simulink model "PeakDetect_500"  (R2018b)
settings: Solver=FixedStepAuto  StartTime=0  StopTime=500*(15e-9)  FixedStep=15e-9  RelTol=1e-3
libraries: simulink x35, hdlsllib x34
(part 2 of 3)

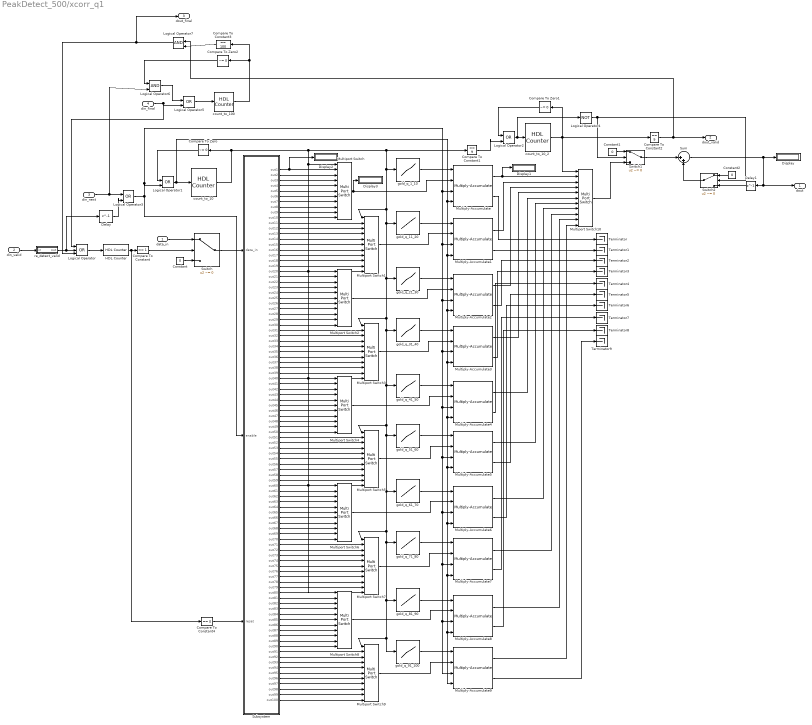
== system PeakDetect_500/xcorr_q1 ==
  data_in : Inport  OutDataTypeStr=fixdt(1,16,15)
  din_valid : Inport  Port=2
  din_next : Inport  Port=3
  din_final : Inport  Port=4
  Compare To Constant : simulink/Logic and Bit Operations/Compare To Constant  relop===  const=1  OutDataTypeStr=boolean
  Compare To Constant1 : simulink/Logic and Bit Operations/Compare To Constant  relop===  const=9  OutDataTypeStr=boolean
  Compare To Constant2 : simulink/Logic and Bit Operations/Compare To Constant  relop===  const=9  OutDataTypeStr=boolean
  Compare To Constant3 : simulink/Logic and Bit Operations/Compare To Constant  relop===  const=100  OutDataTypeStr=boolean
  Compare To Constant4 : simulink/Logic and Bit Operations/Compare To Constant  relop===  const=0  OutDataTypeStr=boolean
  Compare To Zero : simulink/Logic and Bit Operations/Compare To Zero  relop=~=  OutDataTypeStr=boolean
  Compare To Zero1 : simulink/Logic and Bit Operations/Compare To Zero  relop=~=  OutDataTypeStr=boolean
  Compare To Zero2 : simulink/Logic and Bit Operations/Compare To Zero  relop=~=  OutDataTypeStr=boolean
  Constant : Constant  Value=0  OutDataTypeStr=fixdt(1,16,15)  SampleTime=-1
  Constant1 : Constant  Value=0  OutDataTypeStr=Inherit: Inherit via back propagation  SampleTime=-1
  Constant2 : Constant  Value=0  OutDataTypeStr=Inherit: Inherit via back propagation  SampleTime=-1
  Delay : Delay  DelayLength=1
  Delay1 : Delay  DelayLength=1
  Display{,1..3} (4 alike) : Display
  HDL Counter : hdlsllib/Sources/HDL Counter  CountType=Count limited  CountInit=0  CountStep=1  CountMax=2  CountFromType=Initial value  CountFrom=0  CountResetPort=off  CountLoadPort=off  CountEnbPort=on  CountDirPort=off  CountDataType=Unsigned  CountWordLen=8  CountFracLen=0  CountSampTime=1
      settings: SourceProductBaseCode=HD
  Logical Operator : Logic  Operator=OR  Inputs=3  IconShape=distinctive  AllPortsSameDT=off  OutDataTypeStr=boolean
  Logical Operator{1..3,5} (4 alike) : Logic  Operator=OR  IconShape=distinctive  AllPortsSameDT=off  OutDataTypeStr=boolean
  Logical Operator4 : Logic  Operator=NOT  IconShape=distinctive  AllPortsSameDT=off  OutDataTypeStr=boolean
  Logical Operator6 : Logic  IconShape=distinctive  AllPortsSameDT=off  OutDataTypeStr=boolean
  Logical Operator7 : Logic  IconShape=distinctive  AllPortsSameDT=off  OutDataTypeStr=boolean
  Multiply-Accumulate{,1..9} (10 alike) : hdlsllib/HDL Operations/Multiply-Accumulate  opMode=Streaming - using Start and End ports  initValueSetting=Dialog  initValue=0  initValueSetting2=Dialog  initValue2=0  initValueSetting3=Dialog  initValue3=0  num_samples=2  RndMeth2=Floor  RndMeth3=Floor  datatype2=fixdt(1,32,16)  datatype3=Inherit: Inherit via back propagation  validOut=on  endInandOut=off  startOut=off  countOut=on  dim=-1  DoSatur=off  parallel=off
      settings: SourceProductName=HDL Coder  SourceProductBaseCode=HD
  Multiport Switch{,1..9} (10 alike) : MultiPortSwitch  DataPortOrder=Zero-based contiguous  Inputs=10  zeroidx=on  OutDataTypeStr=fixdt(1,16,15)
  Multiport Switch10 : MultiPortSwitch  DataPortOrder=Zero-based contiguous  Inputs=10  zeroidx=on  OutDataTypeStr=fixdt(1,32,16)
  Subsystem : Subsystem
  Sum : Sum  Inputs=|++  OutDataTypeStr=Inherit: Inherit via back propagation
  Switch : Switch  Criteria=u2 ~= 0  OutDataTypeStr=Inherit: Inherit via back propagation
  Switch1 : Switch  Criteria=u2 ~= 0  OutDataTypeStr=Inherit: Inherit via back propagation
  Switch2 : Switch  Criteria=u2 ~= 0  OutDataTypeStr=Inherit: Inherit via back propagation
  Terminator{,1..9} (10 alike) : Terminator
  count_to_10 : hdlsllib/Sources/HDL Counter  CountType=Count limited  CountInit=0  CountStep=1  CountMax=9  CountFromType=Initial value  CountFrom=0  CountResetPort=off  CountLoadPort=off  CountEnbPort=on  CountDirPort=off  CountDataType=Unsigned  CountWordLen=4  CountFracLen=0  CountSampTime=1
      settings: SourceProductBaseCode=HD
  count_to_100 : hdlsllib/Sources/HDL Counter  CountType=Count limited  CountInit=0  CountStep=1  CountMax=100  CountFromType=Initial value  CountFrom=0  CountResetPort=off  CountLoadPort=off  CountEnbPort=on  CountDirPort=off  CountDataType=Unsigned  CountWordLen=8  CountFracLen=0  CountSampTime=1
      settings: SourceProductBaseCode=HD
  count_to_10_2 : hdlsllib/Sources/HDL Counter  CountType=Count limited  CountInit=0  CountStep=1  CountMax=9  CountFromType=Initial value  CountFrom=0  CountResetPort=off  CountLoadPort=off  CountEnbPort=on  CountDirPort=off  CountDataType=Unsigned  CountWordLen=4  CountFracLen=0  CountSampTime=1
      settings: SourceProductBaseCode=HD
  gold_q_11_20 : Lookup_n-D  NumberOfTableDimensions=1  LookupTableObject=''  BreakpointsForDimension1=uint8([0,1,2,3,4,5,6,7,8,9])  BreakpointsForDimension1FirstPoint=10  BreakpointsForDimension2FirstPoint=10  BreakpointsForDimension1Spacing=12  BreakpointsForDimension2Spacing=12  IndexSearchMethod=Evenly spaced points  Table=|  TableDataTypeStr=fixdt(1,16,15)  InterpMethod=Flat  DiagnosticForOutOfRangeInput=Error  InternalRulePriority=Speed  OutDataTypeStr=fixdt(1,16,15)  RndMeth=Simplest  InputSameDT=on
      | -1*[0.236906374990369
      | 0.265062589296935
      | 0.290853922757751
      | 0.306866645010829
      | 0.306877356493505
      | 0.282583044796408
      | 0.237895318583737
      | 0.179451570247324
      | 0.106711739895776
      | 0.0250742736874029]
  gold_q_1_10 : Lookup_n-D  NumberOfTableDimensions=1  LookupTableObject=''  BreakpointsForDimension1=uint8([0,1,2,3,4,5,6,7,8,9])  BreakpointsForDimension1FirstPoint=10  BreakpointsForDimension2FirstPoint=10  BreakpointsForDimension1Spacing=12  BreakpointsForDimension2Spacing=12  IndexSearchMethod=Evenly spaced points  Table=|  TableDataTypeStr=fixdt(1,16,15)  InterpMethod=Flat  DiagnosticForOutOfRangeInput=Error  InternalRulePriority=Speed  OutDataTypeStr=fixdt(1,16,15)  RndMeth=Simplest  InputSameDT=on
      | -1*[0.357169275362262
      | 0.373691122276015
      | 0.363136475782144
      | 0.332586509539436
      | 0.291374087870011
      | 0.249422279627694
      | 0.215579045674242
      | 0.200455944131647
      | 0.201796906991478
      | 0.213779029408702]
  gold_q_21_30 : Lookup_n-D  NumberOfTableDimensions=1  LookupTableObject=''  BreakpointsForDimension1=uint8([0,1,2,3,4,5,6,7,8,9])  BreakpointsForDimension1FirstPoint=10  BreakpointsForDimension2FirstPoint=10  BreakpointsForDimension1Spacing=12  BreakpointsForDimension2Spacing=12  IndexSearchMethod=Evenly spaced points  Table=|  TableDataTypeStr=fixdt(1,16,15)  InterpMethod=Flat  DiagnosticForOutOfRangeInput=Error  InternalRulePriority=Speed  OutDataTypeStr=fixdt(1,16,15)  RndMeth=Simplest  InputSameDT=on
      | -1*[-0.0591515848508664
      | -0.139598314313151
      | -0.210629837752387
      | -0.263713716480122
      | -0.301489962058033
      | -0.328238114626508
      | -0.340130412877520
      | -0.338689881672749
      | -0.326243180584237
      | -0.305614110780615]
  gold_q_31_40 : Lookup_n-D  NumberOfTableDimensions=1  LookupTableObject=''  BreakpointsForDimension1=uint8([0,1,2,3,4,5,6,7,8,9])  BreakpointsForDimension1FirstPoint=10  BreakpointsForDimension2FirstPoint=10  BreakpointsForDimension1Spacing=12  BreakpointsForDimension2Spacing=12  IndexSearchMethod=Evenly spaced points  Table=|  TableDataTypeStr=fixdt(1,16,15)  InterpMethod=Flat  DiagnosticForOutOfRangeInput=Error  InternalRulePriority=Speed  OutDataTypeStr=fixdt(1,16,15)  RndMeth=Simplest  InputSameDT=on
      | -1*[-0.279858098355888
      | -0.247814863771713
      | -0.225446174923891
      | -0.202743193363060
      | -0.186527042991191
      | -0.178781266249413
      | -0.180711431323688
      | -0.192575241083779
      | -0.213551675353351
      | -0.245925394077466]
  gold_q_41_50 : Lookup_n-D  NumberOfTableDimensions=1  LookupTableObject=''  BreakpointsForDimension1=uint8([0,1,2,3,4,5,6,7,8,9])  BreakpointsForDimension1FirstPoint=10  BreakpointsForDimension2FirstPoint=10  BreakpointsForDimension1Spacing=12  BreakpointsForDimension2Spacing=12  IndexSearchMethod=Evenly spaced points  Table=|  TableDataTypeStr=fixdt(1,16,15)  InterpMethod=Flat  DiagnosticForOutOfRangeInput=Error  InternalRulePriority=Speed  OutDataTypeStr=fixdt(1,16,15)  RndMeth=Simplest  InputSameDT=on
      | -1*[-0.273649789754997
      | -0.305507933389466
      | -0.332526349511340
      | -0.349961882407133
      | -0.353614169955030
      | -0.340366684130075
      | -0.308641627170326
      | -0.254460428744123
      | -0.185247665828561
      | -0.110080691949015]
  gold_q_51_60 : Lookup_n-D  NumberOfTableDimensions=1  LookupTableObject=''  BreakpointsForDimension1=uint8([0,1,2,3,4,5,6,7,8,9])  BreakpointsForDimension1FirstPoint=10  BreakpointsForDimension2FirstPoint=10  BreakpointsForDimension1Spacing=12  BreakpointsForDimension2Spacing=12  IndexSearchMethod=Evenly spaced points  Table=|  TableDataTypeStr=fixdt(1,16,15)  InterpMethod=Flat  DiagnosticForOutOfRangeInput=Error  InternalRulePriority=Speed  OutDataTypeStr=fixdt(1,16,15)  RndMeth=Simplest  InputSameDT=on
      | -1*[-0.0297558495000079
      | 0.0499350486257353
      | 0.122950591883728
      | 0.183532283875116
      | 0.226715241693549
      | 0.244522518247979
      | 0.247772413924009
      | 0.223279362418140
      | 0.176793915855740
      | 0.111355596734925]
  gold_q_61_70 : Lookup_n-D  NumberOfTableDimensions=1  LookupTableObject=''  BreakpointsForDimension1=uint8([0,1,2,3,4,5,6,7,8,9])  BreakpointsForDimension1FirstPoint=10  BreakpointsForDimension2FirstPoint=10  BreakpointsForDimension1Spacing=12  BreakpointsForDimension2Spacing=12  IndexSearchMethod=Evenly spaced points  Table=|  TableDataTypeStr=fixdt(1,16,15)  InterpMethod=Flat  DiagnosticForOutOfRangeInput=Error  InternalRulePriority=Speed  OutDataTypeStr=fixdt(1,16,15)  RndMeth=Simplest  InputSameDT=on
      | -1*[0.0312880626224120
      | -0.0580988665112754
      | -0.150830519884918
      | -0.236354458852815
      | -0.321361371110983
      | -0.387151947785857
      | -0.432910784333285
      | -0.454553321854592
      | -0.449340647995131
      | -0.416266380216616]
  gold_q_71_80 : Lookup_n-D  NumberOfTableDimensions=1  LookupTableObject=''  BreakpointsForDimension1=uint8([0,1,2,3,4,5,6,7,8,9])  BreakpointsForDimension1FirstPoint=10  BreakpointsForDimension2FirstPoint=10  BreakpointsForDimension1Spacing=12  BreakpointsForDimension2Spacing=12  IndexSearchMethod=Evenly spaced points  Table=|  TableDataTypeStr=fixdt(1,16,15)  InterpMethod=Flat  DiagnosticForOutOfRangeInput=Error  InternalRulePriority=Speed  OutDataTypeStr=fixdt(1,16,15)  RndMeth=Simplest  InputSameDT=on
      | -1*[-0.356405677154333
      | -0.268905527196357
      | -0.172503144328213
      | -0.0623088722264564
      | 0.0478292512438748
      | 0.147701871156711
      | 0.227579808283800
      | 0.279365016179912
      | 0.297653875710056
      | 0.276310228166542]
  gold_q_81_90 : Lookup_n-D  NumberOfTableDimensions=1  LookupTableObject=''  BreakpointsForDimension1=uint8([0,1,2,3,4,5,6,7,8,9])  BreakpointsForDimension1FirstPoint=10  BreakpointsForDimension2FirstPoint=10  BreakpointsForDimension1Spacing=12  BreakpointsForDimension2Spacing=12  IndexSearchMethod=Evenly spaced points  Table=|  TableDataTypeStr=fixdt(1,16,15)  InterpMethod=Flat  DiagnosticForOutOfRangeInput=Error  InternalRulePriority=Speed  OutDataTypeStr=fixdt(1,16,15)  RndMeth=Simplest  InputSameDT=on
      | -1*[0.222595237130309
      | 0.147485843722747
      | 0.0555170073150737
      | -0.0424496465550990
      | -0.134707118174198
      | -0.210100315272752
      | -0.259403813850479
      | -0.272248751146779
      | -0.259403813850479
      | -0.210100315272752]
  gold_q_91_100 : Lookup_n-D  NumberOfTableDimensions=1  LookupTableObject=''  BreakpointsForDimension1=uint8([0,1,2,3,4,5,6,7,8,9])  BreakpointsForDimension1FirstPoint=10  BreakpointsForDimension2FirstPoint=10  BreakpointsForDimension1Spacing=12  BreakpointsForDimension2Spacing=12  IndexSearchMethod=Evenly spaced points  Table=|  TableDataTypeStr=fixdt(1,16,15)  InterpMethod=Flat  DiagnosticForOutOfRangeInput=Error  InternalRulePriority=Speed  OutDataTypeStr=fixdt(1,16,15)  RndMeth=Simplest  InputSameDT=on
      | -1*[-0.134707118174198
      | -0.0424496465550989
      | 0.0555170073150737
      | 0.147485843722747
      | 0.222595237130309
      | 0.267820298855522
      | 0.290378842162360
      | 0.275261187855880
      | 0.228204197191429
      | 0.153805243290024]
  re_detect_valid : Subsystem
  dout : Outport  OutDataTypeStr=fixdt(1,32,16)
  dout_valid : Outport  Port=2
  dout_final : Outport  Port=3
  wires:
  Subsystem/63(out63) -> Multiport Switch6/4
  Subsystem/83(out83) -> Multiport Switch8/4
  Subsystem/87(out87) -> Multiport Switch8/8
  Subsystem/57(out57) -> Multiport Switch5/8
  count_to_10/1 -> Compare To Zero/1, Multiport Switch8/1, Multiport Switch6/1, Multiport Switch4/1, Multiport Switch2/1, Multiport Switch/1, gold_q_11_20/1, gold_q_21_30/1, gold_q_31_40/1, gold_q_41_50/1, gold_q_51_60/1, gold_q_61_70/1, gold_q_71_80/1, gold_q_81_90/1, gold_q_91_100/1, Multiport Switch9/1, Multiport Switch7/1, Multiport Switch5/1, Multiport Switch3/1, Multiport Switch1/1, gold_q_1_10/1, Compare To Constant1/1
  Subsystem/97(out97) -> Multiport Switch9/8
  Multiply-Accumulate4/1 -> Multiport Switch10/6
  Subsystem/65(out65) -> Multiport Switch6/6
  Subsystem/99(out99) -> Multiport Switch9/10
  Subsystem/73(out73) -> Multiport Switch7/4
  Subsystem/49(out49) -> Multiport Switch4/10
  Multiply-Accumulate/2 -> Terminator/1
  din_final/1 -> Logical Operator/1, Logical Operator5/2
  count_to_10_2/1 -> Compare To Constant2/1, Multiport Switch10/1, Compare To Zero1/1
  Multiport Switch8/1 -> Multiply-Accumulate8/2
  Compare To Constant2/1 -> dout_valid/1, Logical Operator7/1
  Subsystem/61(out61) -> Multiport Switch6/2
  Subsystem/28(out28) -> Multiport Switch2/9
  Subsystem/1(out1) -> Display2/1, Multiport Switch/2
  Multiply-Accumulate6/1 -> Multiport Switch10/8
  Subsystem/100(out100) -> Multiport Switch9/11
  Logical Operator/1 -> HDL Counter/1
  din_valid/1 -> re_detect_valid/1(in)
  Subsystem/68(out68) -> Multiport Switch6/9
  Subsystem/56(out56) -> Multiport Switch5/7
  Subsystem/13(out13) -> Multiport Switch1/4
  Subsystem/67(out67) -> Multiport Switch6/8
  Subsystem/66(out66) -> Multiport Switch6/7
  Logical Operator2/1 -> Logical Operator4/1, count_to_10_2/1
  Constant/1 -> Switch/3
  Compare To Zero/1 -> Logical Operator1/1
  Subsystem/89(out89) -> Multiport Switch8/10
  Multiport Switch5/1 -> Multiply-Accumulate5/2
  Subsystem/29(out29) -> Multiport Switch2/10
  Compare To Constant/1 -> Switch/2
  gold_q_91_100/1 -> Multiply-Accumulate9/1
  Subsystem/52(out52) -> Multiport Switch5/3
  re_detect_valid/1(out) -> Delay/1, Logical Operator/2
  Logical Operator1/1 -> count_to_10/1, Multiply-Accumulate2/4, Multiply-Accumulate9/4, Multiply-Accumulate8/4, Multiply-Accumulate7/4, Multiply-Accumulate6/4, Multiply-Accumulate5/4, Multiply-Accumulate4/4, Multiply-Accumulate3/4, Multiply-Accumulate1/4, Multiply-Accumulate/4
  Subsystem/76(out76) -> Multiport Switch7/7
  Sum/1 -> dout/1, Delay1/1, Display/1
  Logical Operator3/1 -> Subsystem/2(enable), Multiply-Accumulate9/3, Multiply-Accumulate8/3, Multiply-Accumulate7/3, Multiply-Accumulate6/3, Multiply-Accumulate5/3, Multiply-Accumulate4/3, Multiply-Accumulate3/3, Multiply-Accumulate2/3, Multiply-Accumulate1/3, Multiply-Accumulate/3, Logical Operator1/2
  Subsystem/2(out2) -> Multiport Switch/3
  Subsystem/88(out88) -> Multiport Switch8/9
  Subsystem/64(out64) -> Multiport Switch6/5
  Subsystem/41(out41) -> Multiport Switch4/2
  Multiply-Accumulate9/2 -> Terminator9/1
  din_next/1 -> Logical Operator6/2, Logical Operator3/1
  Subsystem/11(out11) -> Multiport Switch1/2
  Subsystem/96(out96) -> Multiport Switch9/7
  Switch1/1 -> Sum/1
  Subsystem/80(out80) -> Multiport Switch7/11
  Subsystem/54(out54) -> Multiport Switch5/5
  Subsystem/82(out82) -> Multiport Switch8/3
  Multiply-Accumulate4/2 -> Terminator4/1
  Subsystem/6(out6) -> Multiport Switch/7
  Subsystem/45(out45) -> Multiport Switch4/6
  Multiport Switch4/1 -> Multiply-Accumulate4/2
  Logical Operator4/1 -> Switch1/2, Switch2/2
  Subsystem/58(out58) -> Multiport Switch5/9
  Subsystem/81(out81) -> Multiport Switch8/2
  Subsystem/44(out44) -> Multiport Switch4/5
  Subsystem/86(out86) -> Multiport Switch8/7
  Subsystem/85(out85) -> Multiport Switch8/6
  Logical Operator5/1 -> count_to_100/1
  Multiport Switch/1 -> Multiply-Accumulate/2, Display3/1
  Subsystem/27(out27) -> Multiport Switch2/8
  gold_q_31_40/1 -> Multiply-Accumulate3/1
  Subsystem/93(out93) -> Multiport Switch9/4
  Compare To Zero1/1 -> Logical Operator2/1
  Subsystem/39(out39) -> Multiport Switch3/10
  Subsystem/84(out84) -> Multiport Switch8/5
  Subsystem/70(out70) -> Multiport Switch6/11
  Subsystem/77(out77) -> Multiport Switch7/8
  Subsystem/62(out62) -> Multiport Switch6/3
  Subsystem/95(out95) -> Multiport Switch9/6
  gold_q_1_10/1 -> Multiply-Accumulate/1
  Compare To Zero2/1 -> Logical Operator6/1
  Multiply-Accumulate1/1 -> Multiport Switch10/3
  Subsystem/47(out47) -> Multiport Switch4/8
  Multiply-Accumulate3/2 -> Terminator3/1
  Subsystem/22(out22) -> Multiport Switch2/3
  Subsystem/92(out92) -> Multiport Switch9/3
  count_to_100/1 -> Compare To Constant3/1, Compare To Zero2/1
  Multiport Switch3/1 -> Multiply-Accumulate3/2
  Subsystem/59(out59) -> Multiport Switch5/10
  Subsystem/9(out9) -> Multiport Switch/10
  Subsystem/5(out5) -> Multiport Switch/6
  gold_q_11_20/1 -> Multiply-Accumulate1/1
  data_in/1 -> Switch/1
  Subsystem/90(out90) -> Multiport Switch8/11
  Subsystem/10(out10) -> Multiport Switch/11
  Subsystem/75(out75) -> Multiport Switch7/6
  Subsystem/18(out18) -> Multiport Switch1/9
  Subsystem/12(out12) -> Multiport Switch1/3
  Subsystem/25(out25) -> Multiport Switch2/6
  Subsystem/43(out43) -> Multiport Switch4/4
  Subsystem/72(out72) -> Multiport Switch7/3
  Subsystem/30(out30) -> Multiport Switch2/11
  Subsystem/8(out8) -> Multiport Switch/9
  Subsystem/60(out60) -> Multiport Switch5/11
  HDL Counter/1 -> Compare To Constant4/1, Compare To Constant/1
  Multiply-Accumulate8/2 -> Terminator8/1
  Subsystem/17(out17) -> Multiport Switch1/8
  Multiply-Accumulate9/1 -> Multiport Switch10/11
  Subsystem/26(out26) -> Multiport Switch2/7
  Subsystem/35(out35) -> Multiport Switch3/6
  Subsystem/24(out24) -> Multiport Switch2/5
  Subsystem/20(out20) -> Multiport Switch1/11
  Subsystem/71(out71) -> Multiport Switch7/2
  Subsystem/78(out78) -> Multiport Switch7/9
  Multiport Switch9/1 -> Multiply-Accumulate9/2
  Subsystem/7(out7) -> Multiport Switch/8
  Subsystem/3(out3) -> Multiport Switch/4
  Subsystem/79(out79) -> Multiport Switch7/10
  Multiport Switch10/1 -> Switch1/3
  Subsystem/15(out15) -> Multiport Switch1/6
  Subsystem/14(out14) -> Multiport Switch1/5
  Multiply-Accumulate/1 -> Display1/1, Multiport Switch10/2
  Subsystem/42(out42) -> Multiport Switch4/3
  Subsystem/16(out16) -> Multiport Switch1/7
  Logical Operator6/1 -> Logical Operator5/1
  Logical Operator7/1 -> dout_final/1, Logical Operator/3
  Subsystem/53(out53) -> Multiport Switch5/4
  Subsystem/37(out37) -> Multiport Switch3/8
  Subsystem/55(out55) -> Multiport Switch5/6
  Subsystem/48(out48) -> Multiport Switch4/9
  Subsystem/4(out4) -> Multiport Switch/5
  Subsystem/50(out50) -> Multiport Switch4/11
  Subsystem/40(out40) -> Multiport Switch3/11
  Switch/1 -> Subsystem/1(data_in)
  Subsystem/19(out19) -> Multiport Switch1/10
  Subsystem/38(out38) -> Multiport Switch3/9
  Subsystem/33(out33) -> Multiport Switch3/4
  Subsystem/46(out46) -> Multiport Switch4/7
  Subsystem/31(out31) -> Multiport Switch3/2
  Subsystem/69(out69) -> Multiport Switch6/10
  Subsystem/94(out94) -> Multiport Switch9/5
  gold_q_71_80/1 -> Multiply-Accumulate7/1
  Subsystem/32(out32) -> Multiport Switch3/3
  Multiply-Accumulate3/1 -> Multiport Switch10/5
  Subsystem/23(out23) -> Multiport Switch2/4
  Multiply-Accumulate2/1 -> Multiport Switch10/4
  Multiport Switch6/1 -> Multiply-Accumulate6/2
  Constant1/1 -> Switch1/1
  Multiply-Accumulate6/2 -> Terminator6/1
  Compare To Constant1/1 -> Logical Operator2/2
  Constant2/1 -> Switch2/1
  Compare To Constant3/1 -> Logical Operator7/2
  gold_q_41_50/1 -> Multiply-Accumulate4/1
  gold_q_21_30/1 -> Multiply-Accumulate2/1
  Multiport Switch2/1 -> Multiply-Accumulate2/2
  Subsystem/21(out21) -> Multiport Switch2/2
  gold_q_61_70/1 -> Multiply-Accumulate6/1
  gold_q_51_60/1 -> Multiply-Accumulate5/1
  Multiply-Accumulate7/1 -> Multiport Switch10/9
  Multiport Switch7/1 -> Multiply-Accumulate7/2
  gold_q_81_90/1 -> Multiply-Accumulate8/1
  Multiport Switch1/1 -> Multiply-Accumulate1/2
  Subsystem/91(out91) -> Multiport Switch9/2
  Multiply-Accumulate5/1 -> Multiport Switch10/7
  Multiply-Accumulate8/1 -> Multiport Switch10/10
  Delay/1 -> Logical Operator3/2
  Delay1/1 -> Switch2/3
  Switch2/1 -> Sum/2
  Subsystem/51(out51) -> Multiport Switch5/2
  Subsystem/36(out36) -> Multiport Switch3/7
  Subsystem/34(out34) -> Multiport Switch3/5
  Compare To Constant4/1 -> Subsystem/3(reset)
  Subsystem/98(out98) -> Multiport Switch9/9
  Multiply-Accumulate5/2 -> Terminator5/1
  Subsystem/74(out74) -> Multiport Switch7/5
  Multiply-Accumulate7/2 -> Terminator7/1
  Multiply-Accumulate1/2 -> Terminator1/1
  Multiply-Accumulate2/2 -> Terminator2/1

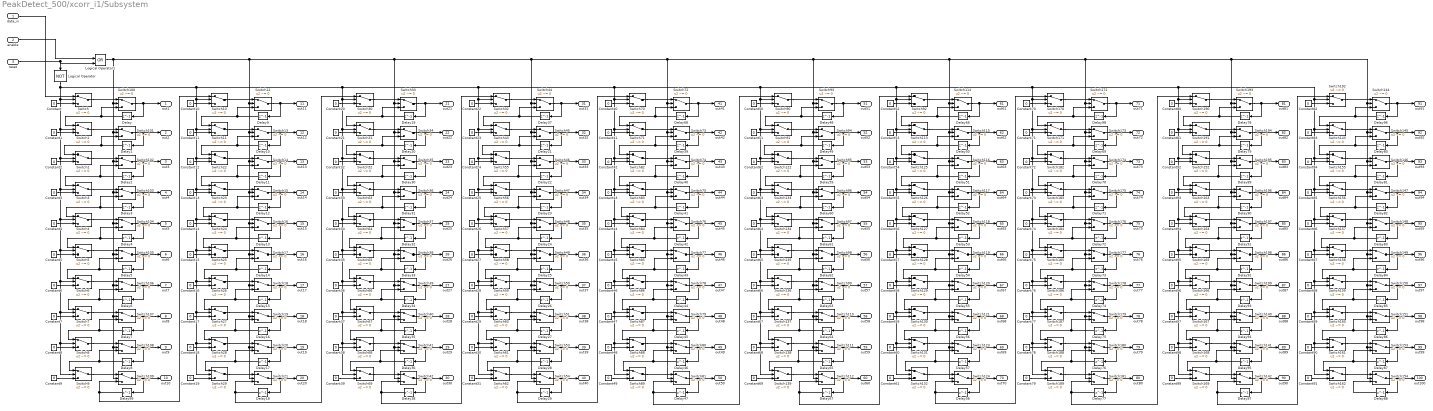
== system PeakDetect_500/xcorr_i1/Subsystem ==
  data_in : Inport  OutDataTypeStr=fixdt(1,16,15)
  enable : Inport  Port=2
  reset : Inport  Port=3
  Constant{,1..99} (100 alike) : Constant  Value=0  OutDataTypeStr=Inherit: Inherit via back propagation  SampleTime=-1
  Delay{,1..99} (100 alike) : Delay  DelayLength=1
  Logical Operator : Logic  Operator=NOT  IconShape=distinctive  AllPortsSameDT=off  OutDataTypeStr=boolean
  Logical Operator1 : Logic  Operator=OR  IconShape=distinctive  AllPortsSameDT=off  OutDataTypeStr=boolean
  Switch{,1..199} (200 alike) : Switch  Criteria=u2 ~= 0  OutDataTypeStr=Inherit: Inherit via back propagation
  out1 : Outport
  out2 : Outport  Port=2
  out3 : Outport  Port=3
  out4 : Outport  Port=4
  out5 : Outport  Port=5
  out6 : Outport  Port=6
  out7 : Outport  Port=7
  out8 : Outport  Port=8
  out9 : Outport  Port=9
  out10 : Outport  Port=10
  out11 : Outport  Port=11
  out12 : Outport  Port=12
  out13 : Outport  Port=13
  out14 : Outport  Port=14
  out15 : Outport  Port=15
  out16 : Outport  Port=16
  out17 : Outport  Port=17
  out18 : Outport  Port=18
  out19 : Outport  Port=19
  out20 : Outport  Port=20
  out21 : Outport  Port=21
  out22 : Outport  Port=22
  out23 : Outport  Port=23
  out24 : Outport  Port=24
  out25 : Outport  Port=25
  out26 : Outport  Port=26
  out27 : Outport  Port=27
  out28 : Outport  Port=28
  out29 : Outport  Port=29
  out30 : Outport  Port=30
  out31 : Outport  Port=31
  out32 : Outport  Port=32
  out33 : Outport  Port=33
  out34 : Outport  Port=34
  out35 : Outport  Port=35
  out36 : Outport  Port=36
  out37 : Outport  Port=37
  out38 : Outport  Port=38
  out39 : Outport  Port=39
  out40 : Outport  Port=40
  out41 : Outport  Port=41
  out42 : Outport  Port=42
  out43 : Outport  Port=43
  out44 : Outport  Port=44
  out45 : Outport  Port=45
  out46 : Outport  Port=46
  out47 : Outport  Port=47
  out48 : Outport  Port=48
  out49 : Outport  Port=49
  out50 : Outport  Port=50
  out51 : Outport  Port=51
  out52 : Outport  Port=52
  out53 : Outport  Port=53
  out54 : Outport  Port=54
  out55 : Outport  Port=55
  out56 : Outport  Port=56
  out57 : Outport  Port=57
  out58 : Outport  Port=58
  out59 : Outport  Port=59
  out60 : Outport  Port=60
  out61 : Outport  Port=61
  out62 : Outport  Port=62
  out63 : Outport  Port=63
  out64 : Outport  Port=64
  out65 : Outport  Port=65
  out66 : Outport  Port=66
  out67 : Outport  Port=67
  out68 : Outport  Port=68
  out69 : Outport  Port=69
  out70 : Outport  Port=70
  out71 : Outport  Port=71
  out72 : Outport  Port=72
  out73 : Outport  Port=73
  out74 : Outport  Port=74
  out75 : Outport  Port=75
  out76 : Outport  Port=76
  out77 : Outport  Port=77
  out78 : Outport  Port=78
  out79 : Outport  Port=79
  out80 : Outport  Port=80
  out81 : Outport  Port=81
  out82 : Outport  Port=82
  out83 : Outport  Port=83
  out84 : Outport  Port=84
  out85 : Outport  Port=85
  out86 : Outport  Port=86
  out87 : Outport  Port=87
  out88 : Outport  Port=88
  out89 : Outport  Port=89
  out90 : Outport  Port=90
  out91 : Outport  Port=91
  out92 : Outport  Port=92
  out93 : Outport  Port=93
  out94 : Outport  Port=94
  out95 : Outport  Port=95
  out96 : Outport  Port=96
  out97 : Outport  Port=97
  out98 : Outport  Port=98
  out99 : Outport  Port=99
  out100 : Outport  Port=100
  wires:
  Delay/1 -> Switch100/3, Switch1/1
  Switch6/1 -> Switch106/1
  Delay8/1 -> Switch108/3, Switch9/1
  Switch3/1 -> Switch103/1
  Switch2/1 -> Switch102/1
  Switch8/1 -> Switch108/1
  Constant2/1 -> Switch2/3
  Constant/1 -> Switch/3
  Switch101/1 -> out2/1, Delay1/1
  Constant6/1 -> Switch6/3
  Constant9/1 -> Switch9/3
  Switch105/1 -> out6/1, Delay5/1
  Switch4/1 -> Switch104/1
  Constant4/1 -> Switch4/3
  Switch100/1 -> out1/1, Delay/1
  Delay7/1 -> Switch107/3, Switch8/1
  Delay3/1 -> Switch103/3, Switch4/1
  Constant8/1 -> Switch8/3
  data_in/1 -> Switch/1
  Switch107/1 -> out8/1, Delay7/1
  Delay2/1 -> Switch102/3, Switch3/1
  Switch103/1 -> Delay3/1, out4/1
  Switch104/1 -> out5/1, Delay4/1
  Constant1/1 -> Switch1/3
  Constant7/1 -> Switch7/3
  Delay6/1 -> Switch106/3, Switch7/1
  Switch102/1 -> Delay2/1, out3/1
  enable/1 -> Logical Operator1/1
  Delay5/1 -> Switch105/3, Switch6/1
  Switch7/1 -> Switch107/1
  Switch109/1 -> Delay99/1, out10/1
  Switch5/1 -> Switch105/1
  Delay4/1 -> Switch104/3, Switch5/1
  Constant5/1 -> Switch5/3
  reset/1 -> Logical Operator1/2, Logical Operator/1
  Switch9/1 -> Switch109/1
  Switch106/1 -> out7/1, Delay6/1
  Constant3/1 -> Switch3/3
  Switch1/1 -> Switch101/1
  Switch/1 -> Switch100/1
  Delay1/1 -> Switch101/3, Switch2/1
  Switch108/1 -> out9/1, Delay8/1
  Delay17/1 -> Switch20/3, Switch29/1
  Delay16/1 -> Switch19/3, Switch28/1
  Delay11/1 -> Switch14/3, Switch23/1
  Constant12/1 -> Switch22/3
  Constant14/1 -> Switch24/3
  Constant19/1 -> Switch29/3
  Switch10/1 -> Switch12/1
  Switch23/1 -> Switch15/1
  Switch17/1 -> out16/1, Delay14/1
  Switch14/1 -> Delay11/1, out13/1
  Switch26/1 -> Switch18/1
  Switch15/1 -> Delay12/1, out14/1
  Switch22/1 -> Switch14/1
  Delay99/1 -> Switch109/3, Switch10/1
  Constant11/1 -> Switch11/3
  Switch11/1 -> Switch13/1
  Constant10/1 -> Switch10/3
  Switch18/1 -> out17/1, Delay15/1
  Switch24/1 -> Switch16/1
  Switch12/1 -> out11/1, Delay9/1
  Constant13/1 -> Switch23/3
  Switch28/1 -> Switch20/1
  Switch16/1 -> out15/1, Delay13/1
  Switch25/1 -> Switch17/1
  Switch20/1 -> out19/1, Delay17/1
  Switch21/1 -> Delay18/1, out20/1
  Constant18/1 -> Switch28/3
  Switch13/1 -> out12/1, Delay10/1
  Switch27/1 -> Switch19/1
  Delay15/1 -> Switch18/3, Switch27/1
  Constant16/1 -> Switch26/3
  Delay13/1 -> Switch16/3, Switch25/1
  Constant15/1 -> Switch25/3
  Delay12/1 -> Switch15/3, Switch24/1
  Delay10/1 -> Switch13/3, Switch22/1
  Delay9/1 -> Switch12/3, Switch11/1
  Constant17/1 -> Switch27/3
  Delay14/1 -> Switch17/3, Switch26/1
  Switch19/1 -> out18/1, Delay16/1
  Switch29/1 -> Switch21/1
  Delay34/1 -> Switch39/3, Switch67/1
  Delay36/1 -> Switch41/3, Switch69/1
  Constant21/1 -> Switch31/3
  Delay30/1 -> Switch35/3, Switch63/1
  Constant34/1 -> Switch64/3
  Delay25/1 -> Switch49/3, Switch59/1
  Switch67/1 -> Switch40/1
  Switch57/1 -> Switch48/1
  Switch51/1 -> out38/1, Delay27/1
  Switch50/1 -> out37/1, Delay26/1
  Constant24/1 -> Switch55/3
  Switch35/1 -> Delay30/1, out23/1
  Switch39/1 -> out27/1, Delay34/1
  Switch56/1 -> Switch47/1
  Switch42/1 -> Delay38/1, out30/1
  Delay31/1 -> Switch36/3, Switch64/1
  Switch63/1 -> Switch36/1
  Delay27/1 -> Switch51/3, Switch61/1
  Constant39/1 -> Switch69/3
  Switch49/1 -> out36/1, Delay25/1
  Constant29/1 -> Switch60/3
  Switch46/1 -> Delay22/1, out33/1
  Constant25/1 -> Switch56/3
  Switch38/1 -> out26/1, Delay33/1
  Switch47/1 -> Delay23/1, out34/1
  Switch66/1 -> Switch39/1
  Delay35/1 -> Switch40/3, Switch68/1
  Switch64/1 -> Switch37/1
  Switch62/1 -> Switch54/1
  Switch31/1 -> Switch34/1
  Switch33/1 -> out21/1, Delay19/1
  Switch60/1 -> Switch51/1
  Switch58/1 -> Switch49/1
  Constant23/1 -> Switch43/3
  Switch59/1 -> Switch50/1
  Switch52/1 -> Switch35/1
  Constant22/1 -> Switch32/3
  Constant36/1 -> Switch66/3
  Delay38/1 -> Switch42/3, Switch32/1
  Switch41/1 -> out29/1, Delay36/1
  Switch65/1 -> Switch38/1
  Delay28/1 -> Switch53/3, Switch62/1
  Switch37/1 -> out25/1, Delay32/1
  Switch48/1 -> out35/1, Delay24/1
  Constant28/1 -> Switch59/3
  Constant31/1 -> Switch62/3
  Delay32/1 -> Switch37/3, Switch65/1
  Delay37/1 -> Switch44/3, Switch43/1
  Switch30/1 -> Switch33/1
  Switch43/1 -> Switch45/1
  Delay21/1 -> Switch45/3, Switch55/1
  Switch32/1 -> Switch44/1
  Switch44/1 -> out31/1, Delay37/1
  Constant33/1 -> Switch63/3
  Switch61/1 -> Switch53/1
  Switch68/1 -> Switch41/1
  Switch45/1 -> out32/1, Delay21/1
  Delay24/1 -> Switch48/3, Switch58/1
  Delay26/1 -> Switch50/3, Switch60/1
  Switch54/1 -> Delay29/1, out40/1
  Constant20/1 -> Switch30/3
  Switch36/1 -> Delay31/1, out24/1
  Constant32/1 -> Switch52/3
  Constant30/1 -> Switch61/3
  Delay18/1 -> Switch21/3, Switch30/1
  Switch55/1 -> Switch46/1
  Constant26/1 -> Switch57/3
  Constant38/1 -> Switch68/3
  Switch34/1 -> out22/1, Delay20/1
  Constant27/1 -> Switch58/3
  Constant35/1 -> Switch65/3
  Delay20/1 -> Switch34/3, Switch52/1
  Delay19/1 -> Switch33/3, Switch31/1
  Constant37/1 -> Switch67/3
  Delay33/1 -> Switch38/3, Switch66/1
  Switch40/1 -> out28/1, Delay35/1
  Switch69/1 -> Switch42/1
  Delay23/1 -> Switch47/3, Switch57/1
  Switch53/1 -> out39/1, Delay28/1
  Delay22/1 -> Switch46/3, Switch56/1
  Delay65/1 -> Switch111/3, Switch139/1
  Constant54/1 -> Switch125/3
  Switch88/1 -> Switch80/1
  Switch127/1 -> Switch118/1
  Constant60/1 -> Switch131/3
  Delay49/1 -> Switch94/3, Switch122/1
  Switch92/1 -> Switch114/1
  Constant67/1 -> Switch137/3
  Switch116/1 -> Delay51/1, out63/1
  Delay50/1 -> Switch115/3, Switch125/1
  Switch74/1 -> Delay40/1, out43/1
  Constant56/1 -> Switch127/3
  Delay66/1 -> Switch114/3, Switch113/1
  Switch75/1 -> Delay41/1, out44/1
  Delay52/1 -> Switch117/3, Switch127/1
  Switch90/1 -> Switch93/1
  Delay40/1 -> Switch74/3, Switch83/1
  Switch114/1 -> out61/1, Delay66/1
  Switch136/1 -> Switch99/1
  Constant44/1 -> Switch84/3
  Switch120/1 -> out67/1, Delay55/1
  Switch135/1 -> Switch98/1
  Switch91/1 -> Switch94/1
  Switch115/1 -> out62/1, Delay50/1
  Constant45/1 -> Switch85/3
  Constant55/1 -> Switch126/3
  Constant41/1 -> Switch71/3
  Delay62/1 -> Switch98/3, Switch136/1
  Delay29/1 -> Switch54/3, Switch70/1
  Switch78/1 -> out47/1, Delay44/1
  Constant65/1 -> Switch135/3
  Constant61/1 -> Switch132/3
  Switch121/1 -> out68/1, Delay56/1
  Constant48/1 -> Switch88/3
  Switch137/1 -> Switch110/1
  Constant40/1 -> Switch70/3
  Constant46/1 -> Switch86/3
  Delay44/1 -> Switch78/3, Switch87/1
  Switch86/1 -> Switch78/1
  Switch113/1 -> Switch115/1
  Constant52/1 -> Switch92/3
  Constant69/1 -> Switch139/3
  Delay56/1 -> Switch121/3, Switch131/1
  Delay53/1 -> Switch118/3, Switch128/1
  Switch76/1 -> out45/1, Delay42/1
  Switch110/1 -> out58/1, Delay64/1
  Constant66/1 -> Switch136/3
  Switch118/1 -> out65/1, Delay53/1
  Delay39/1 -> Switch73/3, Switch82/1
  Switch99/1 -> out57/1, Delay63/1
  Delay60/1 -> Switch96/3, Switch134/1
  Delay68/1 -> Switch72/3, Switch71/1
  Switch94/1 -> out52/1, Delay49/1
  Switch139/1 -> Switch112/1
  Delay63/1 -> Switch99/3, Switch137/1
  Switch79/1 -> out48/1, Delay45/1
  Constant57/1 -> Switch128/3
  Switch82/1 -> Switch74/1
  Switch111/1 -> out59/1, Delay65/1
  Switch124/1 -> Delay58/1, out70/1
  Constant63/1 -> Switch133/3
  Delay61/1 -> Switch97/3, Switch135/1
  Switch123/1 -> out69/1, Delay57/1
  Switch117/1 -> Delay52/1, out64/1
  Switch129/1 -> Switch120/1
  Delay46/1 -> Switch80/3, Switch89/1
  Switch70/1 -> Switch72/1
  Switch77/1 -> out46/1, Delay43/1
  Switch72/1 -> out41/1, Delay68/1
  Switch133/1 -> Switch96/1
  Delay64/1 -> Switch110/3, Switch138/1
  Delay43/1 -> Switch77/3, Switch86/1
  Switch125/1 -> Switch116/1
  Constant64/1 -> Switch134/3
  Switch130/1 -> Switch121/1
  Constant51/1 -> Switch91/3
  Switch112/1 -> Delay67/1, out60/1
  Switch119/1 -> out66/1, Delay54/1
  Switch87/1 -> Switch79/1
  Delay59/1 -> Switch95/3, Switch133/1
  Switch73/1 -> out42/1, Delay39/1
  Delay42/1 -> Switch76/3, Switch85/1
  Switch122/1 -> Switch95/1
  Constant68/1 -> Switch138/3
  Switch84/1 -> Switch76/1
  Switch98/1 -> out56/1, Delay62/1
  Switch85/1 -> Switch77/1
  Switch95/1 -> Delay59/1, out53/1
  Switch71/1 -> Switch73/1
  Constant42/1 -> Switch82/3
  Switch134/1 -> Switch97/1
  Constant53/1 -> Switch113/3
  Delay57/1 -> Switch123/3, Switch132/1
  Constant47/1 -> Switch87/3
  Delay45/1 -> Switch79/3, Switch88/1
  Switch81/1 -> Delay47/1, out50/1
  Switch93/1 -> out51/1, Delay48/1
  Switch132/1 -> Switch124/1
  Switch97/1 -> out55/1, Delay61/1
  Delay54/1 -> Switch119/3, Switch129/1
  Switch138/1 -> Switch111/1
  Delay47/1 -> Switch81/3, Switch90/1
  Switch83/1 -> Switch75/1
  Switch131/1 -> Switch123/1
  Switch126/1 -> Switch117/1
  Delay67/1 -> Switch112/3, Switch92/1
  Switch128/1 -> Switch119/1
  Constant50/1 -> Switch90/3
  Constant43/1 -> Switch83/3
  Delay51/1 -> Switch116/3, Switch126/1
  Constant62/1 -> Switch122/3
  Constant49/1 -> Switch89/3
  Constant58/1 -> Switch129/3
  Switch89/1 -> Switch81/1
  Delay55/1 -> Switch120/3, Switch130/1
  Switch96/1 -> Delay60/1, out54/1
  Delay41/1 -> Switch75/3, Switch84/1
  Switch80/1 -> out49/1, Delay46/1
  Delay48/1 -> Switch93/3, Switch91/1
  Constant59/1 -> Switch130/3
  Delay72/1 -> Switch176/3, Switch185/1
  Constant78/1 -> Switch188/3
  Switch173/1 -> out72/1, Delay69/1
  Constant91/1 -> Switch162/3
  Constant95/1 -> Switch165/3
  Switch180/1 -> out79/1, Delay76/1
  Switch163/1 -> Switch196/1
  Switch199/1 -> out87/1, Delay93/1
  Switch161/1 -> Switch153/1
  Switch183/1 -> Switch175/1
  Switch149/1 -> out96/1, Delay84/1
  Switch164/1 -> Switch197/1
  Constant80/1 -> Switch190/3
  Constant82/1 -> Switch192/3
  Constant92/1 -> Switch152/3
  Switch143/1 -> Switch145/1
  Switch165/1 -> Switch198/1
  Switch181/1 -> Delay77/1, out80/1
  Switch195/1 -> Delay89/1, out83/1
  Delay89/1 -> Switch195/3, Switch163/1
  Switch185/1 -> Switch177/1
  Constant71/1 -> Switch171/3
  Switch145/1 -> out92/1, Delay80/1
  Switch171/1 -> Switch173/1
  Switch191/1 -> Switch194/1
  Constant73/1 -> Switch183/3
  Constant83/1 -> Switch143/3
  Switch194/1 -> out82/1, Delay79/1
  Constant85/1 -> Switch156/3
  Constant96/1 -> Switch166/3
  Constant86/1 -> Switch157/3
  Delay94/1 -> Switch140/3, Switch168/1
  Switch176/1 -> out75/1, Delay72/1
  Constant79/1 -> Switch189/3
  Switch187/1 -> Switch179/1
  Delay58/1 -> Switch124/3, Switch170/1
  Switch189/1 -> Switch181/1
  Delay77/1 -> Switch181/3, Switch190/1
  Delay98/1 -> Switch172/3, Switch171/1
  Switch150/1 -> out97/1, Delay85/1
  Switch169/1 -> Switch142/1
  Constant89/1 -> Switch160/3
  Switch152/1 -> Switch195/1
  Switch168/1 -> Switch141/1
  Switch196/1 -> Delay90/1, out84/1
  Switch140/1 -> out88/1, Delay94/1
  Switch146/1 -> Delay81/1, out93/1
  Switch159/1 -> Switch150/1
  Switch172/1 -> out71/1, Delay98/1
  Constant72/1 -> Switch182/3
  Delay74/1 -> Switch178/3, Switch187/1
  Delay71/1 -> Switch175/3, Switch184/1
  Delay78/1 -> Switch193/3, Switch191/1
  Constant94/1 -> Switch164/3
  Switch167/1 -> Switch140/1
  Delay97/1 -> Switch142/3, Switch192/1
  Delay84/1 -> Switch149/3, Switch159/1
  Logical Operator/1 -> Switch162/2, Switch161/2, Switch160/2, Switch159/2, Switch158/2, Switch157/2, Switch156/2, Switch155/2, Switch143/2, Switch192/2, Switch169/2, Switch168/2, Switch167/2, Switch166/2, Switch165/2, Switch164/2, Switch163/2, Switch152/2, Switch191/2, Switch190/2, Switch189/2, Switch188/2, Switch187/2, Switch186/2, Switch185/2, Switch184/2, Switch183/2, Switch182/2, Switch171/2, Switch170/2, Switch132/2, Switch131/2, Switch130/2, Switch129/2, Switch128/2, Switch127/2, Switch126/2, Switch125/2, Switch113/2, Switch92/2, Switch139/2, Switch138/2, Switch137/2, Switch136/2, Switch135/2, Switch134/2, Switch133/2, Switch122/2, Switch91/2, Switch90/2, Switch89/2, Switch88/2, Switch87/2, Switch86/2, Switch85/2, Switch84/2, Switch83/2, Switch82/2, Switch71/2, Switch70/2, Switch62/2, Switch61/2, Switch60/2, Switch59/2, Switch58/2, Switch57/2, Switch56/2, Switch55/2, Switch43/2, Switch32/2, Switch69/2, Switch68/2, Switch67/2, Switch66/2, Switch65/2, Switch64/2, Switch63/2, Switch52/2, Switch31/2, Switch30/2, Switch29/2, Switch28/2, Switch27/2, Switch26/2, Switch25/2, Switch24/2, Switch23/2, Switch22/2, Switch11/2, Switch10/2, Switch9/2, Switch8/2, Switch7/2, Switch6/2, Switch5/2, Switch4/2, Switch3/2, Switch2/2, Switch1/2, Switch/2
  Delay75/1 -> Switch179/3, Switch188/1
  Constant70/1 -> Switch170/3
  Switch177/1 -> out76/1, Delay73/1
  Switch147/1 -> Delay82/1, out94/1
  Switch154/1 -> Delay88/1, out100/1
  Switch179/1 -> out78/1, Delay75/1
  Delay73/1 -> Switch177/3, Switch186/1
  Constant93/1 -> Switch163/3
  Delay87/1 -> Switch153/3, Switch162/1
  Logical Operator1/1 -> Switch41/2, Switch42/2, Switch40/2, Switch39/2, Switch38/2, Switch37/2, Switch36/2, Switch35/2, Switch34/2, Switch33/2, Switch53/2, Switch54/2, Switch51/2, Switch50/2, Switch49/2, Switch48/2, Switch47/2, Switch46/2, Switch45/2, Switch44/2, Switch111/2, Switch112/2, Switch110/2, Switch99/2, Switch98/2, Switch97/2, Switch96/2, Switch95/2, Switch94/2, Switch93/2, Switch123/2, Switch124/2, Switch121/2, Switch120/2, Switch119/2, Switch118/2, Switch117/2, Switch116/2, Switch115/2, Switch114/2, Switch180/2, Switch181/2, Switch179/2, Switch178/2, Switch177/2, Switch176/2, Switch175/2, Switch174/2, Switch173/2, Switch172/2, Switch141/2, Switch142/2, Switch140/2, Switch199/2, Switch198/2, Switch197/2, Switch196/2, Switch195/2, Switch194/2, Switch193/2, Switch153/2, Switch154/2, Switch151/2, Switch150/2, Switch149/2, Switch148/2, Switch147/2, Switch146/2, Switch145/2, Switch144/2, Switch80/2, Switch81/2, Switch79/2, Switch78/2, Switch77/2, Switch76/2, Switch75/2, Switch74/2, Switch73/2, Switch72/2, Switch20/2, Switch21/2, Switch19/2, Switch18/2, Switch17/2, Switch16/2, Switch15/2, Switch14/2, Switch13/2, Switch12/2, Switch108/2, Switch109/2, Switch107/2, Switch106/2, Switch105/2, Switch104/2, Switch103/2, Switch102/2, Switch101/2, Switch100/2
  Constant98/1 -> Switch168/3
  Switch175/1 -> Delay71/1, out74/1
  Delay76/1 -> Switch180/3, Switch189/1
  Delay83/1 -> Switch148/3, Switch158/1
  Constant99/1 -> Switch169/3
  Delay88/1 -> Switch154/3
  Switch193/1 -> out81/1, Delay78/1
  Switch190/1 -> Switch193/1
  Delay69/1 -> Switch173/3, Switch182/1
  Switch170/1 -> Switch172/1
  Switch155/1 -> Switch146/1
  Switch142/1 -> Delay97/1, out90/1
  Constant81/1 -> Switch191/3
  Switch160/1 -> Switch151/1
  Switch162/1 -> Switch154/1
  Switch158/1 -> Switch149/1
  Switch184/1 -> Switch176/1
  Constant74/1 -> Switch184/3
  Delay81/1 -> Switch146/3, Switch156/1
  Switch153/1 -> out99/1, Delay87/1
  Switch198/1 -> out86/1, Delay92/1
  Constant77/1 -> Switch187/3
  Switch197/1 -> out85/1, Delay91/1
  Delay95/1 -> Switch141/3, Switch169/1
  Constant84/1 -> Switch155/3
  Constant75/1 -> Switch185/3
  Delay93/1 -> Switch199/3, Switch167/1
  Delay79/1 -> Switch194/3, Switch152/1
  Constant87/1 -> Switch158/3
  Switch188/1 -> Switch180/1
  Switch157/1 -> Switch148/1
  Switch174/1 -> Delay70/1, out73/1
  Delay70/1 -> Switch174/3, Switch183/1
  Switch156/1 -> Switch147/1
  Switch144/1 -> out91/1, Delay96/1
  Constant76/1 -> Switch186/3
  Switch141/1 -> out89/1, Delay95/1
  Delay82/1 -> Switch147/3, Switch157/1
  Delay85/1 -> Switch150/3, Switch160/1
  Delay91/1 -> Switch197/3, Switch165/1
  Switch192/1 -> Switch144/1
  Constant97/1 -> Switch167/3
  Constant88/1 -> Switch159/3
  Switch182/1 -> Switch174/1
  Constant90/1 -> Switch161/3
  Delay90/1 -> Switch196/3, Switch164/1
  Delay86/1 -> Switch151/3, Switch161/1
  Delay96/1 -> Switch144/3, Switch143/1
  Switch186/1 -> Switch178/1
  Switch166/1 -> Switch199/1
  Delay92/1 -> Switch198/3, Switch166/1
  Delay80/1 -> Switch145/3, Switch155/1
  Switch178/1 -> out77/1, Delay74/1
  Switch151/1 -> out98/1, Delay86/1
  Switch148/1 -> out95/1, Delay83/1

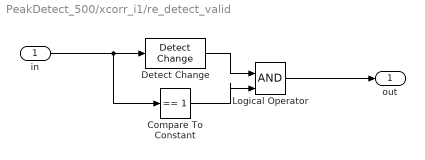
== system PeakDetect_500/xcorr_i1/re_detect_valid ==
  in : Inport  OutDataTypeStr=boolean
  Compare To Constant : simulink/Logic and Bit Operations/Compare To Constant  relop===  const=1  OutDataTypeStr=boolean
  Detect Change : simulink/Logic and Bit Operations/Detect Change  vinit=0  OutDataTypeStr=boolean
  Logical Operator : Logic  IconShape=distinctive  AllPortsSameDT=off  OutDataTypeStr=boolean
  out : Outport  OutDataTypeStr=boolean
  wires:
  Logical Operator/1 -> out/1
  Compare To Constant/1 -> Logical Operator/2
  Detect Change/1 -> Logical Operator/1
  in/1 -> Compare To Constant/1, Detect Change/1
